simulink model "controlador"  (R2023b)
settings: Solver=VariableStepAuto  StartTime=0.0  StopTime=0.008  RelTol=1e-3
values from neighbouring files (symbols this model uses):
  denG = [L*C1 L/R 1]    [SimCONTROL-plantaMAT.m]
  gainI = controlador_pid.Ki    [SimCONTROL-plantaARX.m]    (also in SimCONTROL-plantaMAT.m)
  gainP = controlador_pid.Kp    [SimCONTROL-plantaARX.m]    (also in SimCONTROL-plantaMAT.m)
  numG = U1    (= 30)    [SimCONTROL-plantaMAT.m]
settings Model: Creator=luisf  LastModifiedBy=luisf
settings RTWCC: GenCodeOnly=on

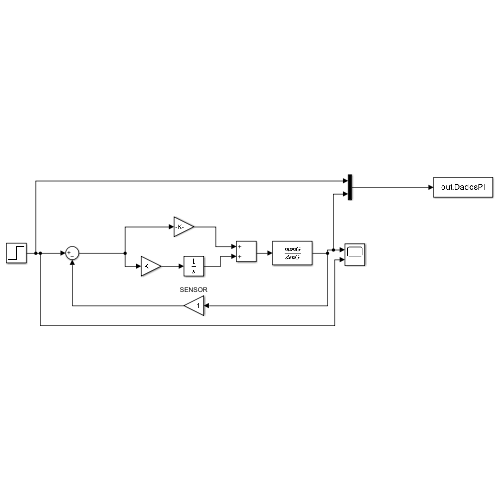
[thumbnail: Simulink's stored preview of the top-level diagram]
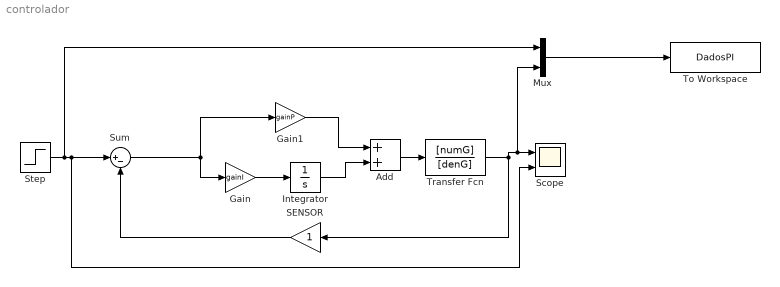
== system controlador ==
  Add : Sum
  Gain : Gain  Gain=gainI
  Gain1 : Gain  Gain=gainP
  Integrator : Integrator
  Mux : Mux  Inputs=2
  SENSOR : Gain
  Scope : Scope  NumInputPorts=2
  Step : Step  Time=0.001  SampleTime=0
  Sum : Sum  Inputs=|+-
  To Workspace : ToWorkspace  VariableName=DadosPI  SampleTime=-1
  Transfer Fcn : TransferFcn  Numerator=[numG]  Denominator=[denG]
  wires:
  Step/1 -> Mux/1, Scope/2, Sum/1
  Sum/1 -> Gain1/1, Gain/1
  Gain1/1 -> Add/1
  Gain/1 -> Integrator/1
  Integrator/1 -> Add/2
  Add/1 -> Transfer Fcn/1
  Transfer Fcn/1 -> SENSOR/1, Mux/2, Scope/1
  Mux/1 -> To Workspace/1
  SENSOR/1 -> Sum/2
